simulink model "model1"  (Simulink 6.4)
settings: Solver=ode45  StartTime=0.0  StopTime=10.0  RelTol=1e-3
undefined symbols (not defined in the file): MinMax, tllib
settings Model: LastModifiedBy=juergens

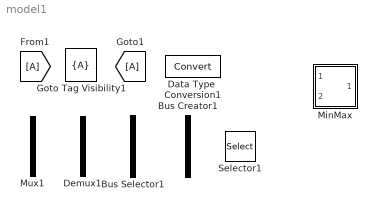
== system model1 ==
  Bus Creator1 : BusCreator  Inputs=2
  Bus Selector1 : BusSelector  OutputSignals=empty
  Data Type  Conversion1 : DataTypeConversion  OutDataTypeMode=double  SaturateOnIntegerOverflow=on  RndMeth=Zero
  Demux1 : Demux  Outputs=2
  Goto Tag Visibility1 : GotoTagVisibility
  MinMax : Subsystem  AncestorBlock=tllib/MinMax  mask(TL_MinMax){data=struct('comment',struct('text','','placement',1),'inputs','2','logdata',struct('maxnumvals',inf,'plotchannels',[],'loggingmode',3,'channels',1),'output',struct('variable','','description','','name','$S_$B','width',1,'address','','max',NaN,'min',NaN,'class','default','type','Int16','scaling','','lsb',1,'offset',0,'arb',0,'freeze',1,'unit','','autoscalingmode',1,'lowerheadroom',1,'upperheadroom',1,'headroomunit','bit','keepdatatype',1,'checkmin',0,'checkmax',0,'castoutput',0,'show',0),'inheritscaling',0,'function','min','scalingvalid',0,'date',730486), lower_limit=, upper_limit=, flp_block=built-in/MinMax, slscaleparams=, help=}
      mask help:
      | TargetLink MinMax block:
      | Output is the minimum/maximum of all inputs.
      mask init:
      | hBlock = gcbh;
      | blockPath = getfullname(hBlock);
      | set_param(hBlock, 'flp_block', flp_block);
      | tlData = eval(data);
      | mmObj = get_param([blockPath, '/MinMax'], 'Object');
      | mmObj.Function = tlData.function;
      | try
      |     mmObj.InputSameDT = 'off';
      | end
      | dispstr = tlData.function;
      | 
      | % adapt block content if necessary
      | blkObj = get_param(hBlock, 'Object');
      | requiredNumInputs = eval(tlData.inputs);
      | currentNumInputs = blkObj.Ports(1);
      | if requiredNumInputs ~= currentNumInputs
      |     % remove superflous inputs
      |     if requiredNumInputs < currentNumInputs
      |         for m = (requiredNumInputs + 1):currentNumInputs
      |             inportObj = get_param(get_param([blockPath, '/In', sprintf('%d', m)], 'Handle'), 'Object');
      |             delete_line(inportObj.LineHandles.Outport);
      |             inportObj.delete;
      |             clear inportObj
      |         end
      |     end
      |     % set parameters of minmax block
      |     mmObj.Inputs = tlData.inputs;
      |     mmObj.Position = [100, 40, 140, (requiredNumInputs * 20 + 50)];
      |     % rearrange existing inports / insert new inports
      |     for m = 1:requiredNumInputs
      |         portPos = get_param(mmObj.PortHandles.Inport(m),'Position');
      |         inportName = [blockPath, '/In', sprintf('%d', m)];
      |         inportPos = [30, portPos(2)-7, 60, (portPos(2) + 7)];
      |         if m <= currentNumInputs
      |             set_param(inportName, 'Position', inportPos);
      |         else
      |             add_block('built-in/Inport', inportName, 'Position', inportPos);
      |             add_line(mmObj.Parent, sprintf('In%d/1', m), sprintf('MinMax/%d', m));
      |         end
      |     end	
      |     clear m mmObj portPos inportName inportPos
      | end
      | clear hBlock blockPath tlData blkObj requiredNumInputs currentNumInputs;
      settings: CopyFcn=if exist('tl_reset_reviewflag') == 2, tl_reset_reviewflag(gcbh); end  DeleteFcn=delete_tlblock(gcbh)  NameChangeFcn=rename_tlblock(gcbh);  OpenFcn=dstabdlg('create','tl_minmax_dlg',gcbh);
      mask Help: eval(['tl_online_help(''Topic'',''',get_param(gcbh,'MaskType'),''')'])
      mask Display:
      | plot([-0.05,1.05],[0.01,0.01],[-0.05,1.05],[0.99,0.99]);
      | disp(dispstr);
  Mux1 : Mux  Inputs=2
  Selector1 : Selector  Elements=[1 3]  InputPortWidth=3

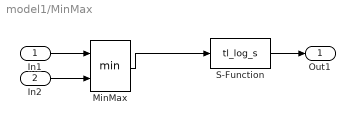
== system model1/MinMax ==
  In1 : Inport
  In2 : Inport  Port=2
  MinMax : MinMax  Inputs=2  SaturateOnIntegerOverflow=on
  S-Function : S-Function  FunctionName=tl_log_s  Parameters=data
  Out1 : Outport
  wires:
  MinMax/1 -> S-Function/1
  In1/1 -> MinMax/1
  S-Function/1 -> Out1/1
  In2/1 -> MinMax/2
